simulink model "TST_PIntkVUs_VD"  (R2016b)
settings: Solver=FixedStepDiscrete  StartTime=0.0  StopTime=simTime  FixedStep=sampleTime  RelTol=1e-3
values from neighbouring files (symbols this model uses):
  testCase = 1    [initTST_PIntkVUs_VD_001.m]    (also in initTST_PIntkVUs_VD_002.m = 2; initTST_PIntkVUs_VD_003.m = 3)
libraries: simulink x7, UnitTest_Lib x3
settings Model: Creator=zhengjinyan  LastModifiedBy=zhengjinyan
settings DebuggingCC: SignalRangeChecking=error

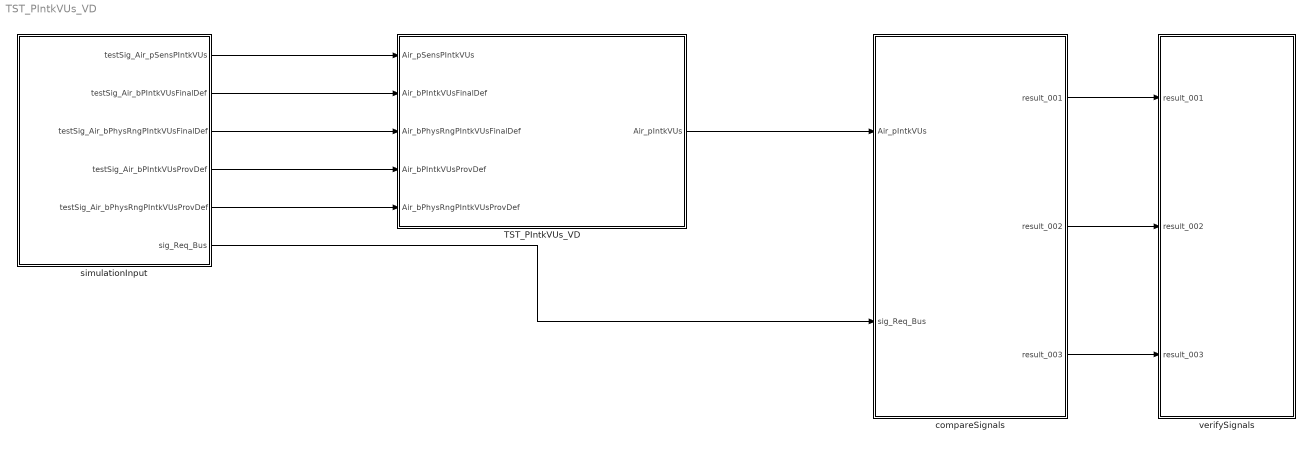
== system TST_PIntkVUs_VD ==
  TST_PIntkVUs_VD : Subsystem
  compareSignals : Subsystem
  simulationInput : Subsystem
  verifySignals : Subsystem
  wires:
  simulationInput/1(testSig_Air_pSensPIntkVUs) -> TST_PIntkVUs_VD/1(Air_pSensPIntkVUs)
  simulationInput/2(testSig_Air_bPIntkVUsFinalDef) -> TST_PIntkVUs_VD/2(Air_bPIntkVUsFinalDef)
  simulationInput/3(testSig_Air_bPhysRngPIntkVUsFinalDef) -> TST_PIntkVUs_VD/3(Air_bPhysRngPIntkVUsFinalDef)
  simulationInput/4(testSig_Air_bPIntkVUsProvDef) -> TST_PIntkVUs_VD/4(Air_bPIntkVUsProvDef)
  simulationInput/5(testSig_Air_bPhysRngPIntkVUsProvDef) -> TST_PIntkVUs_VD/5(Air_bPhysRngPIntkVUsProvDef)
  TST_PIntkVUs_VD/1(Air_pIntkVUs) -> compareSignals/1(Air_pIntkVUs)
  simulationInput/6(sig_Req_Bus) -> compareSignals/2(sig_Req_Bus)
  compareSignals/1(result_001) -> verifySignals/1(result_001)
  compareSignals/2(result_002) -> verifySignals/2(result_002)
  compareSignals/3(result_003) -> verifySignals/3(result_003)

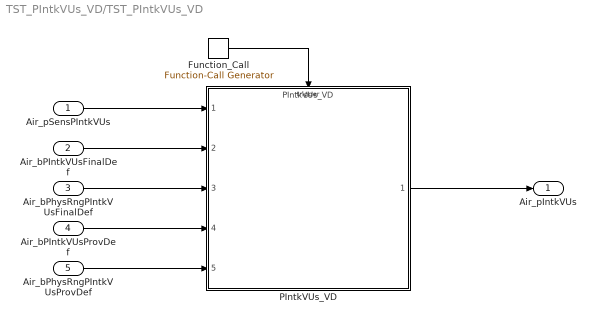
== system TST_PIntkVUs_VD/TST_PIntkVUs_VD ==
  Air_pSensPIntkVUs : Inport
  Air_bPIntkVUsFinalDef : Inport  Port=2
  Air_bPhysRngPIntkVUsFinalDef : Inport  Port=3
  Air_bPIntkVUsProvDef : Inport  Port=4
  Air_bPhysRngPIntkVUsProvDef : Inport  Port=5
  Function_Call : simulink/Ports & Subsystems/Function-Call Generator  sample_time=sampleTime  numberOfIterations=1
  PIntkVUs_VD : ModelReference  ModelNameDialog=PIntkVUs_VD  SimulationMode=Normal  ModelReferenceVersion=1.31  TriggerPortName=function  TriggerPortTriggerType=function-call  TriggerPortStatesWhenEnabling=held
  Air_pIntkVUs : Outport
  wires:
  Function_Call/1 -> PIntkVUs_VD/Trigger
  Air_pSensPIntkVUs/1 -> PIntkVUs_VD/1
  Air_bPIntkVUsFinalDef/1 -> PIntkVUs_VD/2
  Air_bPhysRngPIntkVUsFinalDef/1 -> PIntkVUs_VD/3
  Air_bPIntkVUsProvDef/1 -> PIntkVUs_VD/4
  Air_bPhysRngPIntkVUsProvDef/1 -> PIntkVUs_VD/5
  PIntkVUs_VD/1 -> Air_pIntkVUs/1

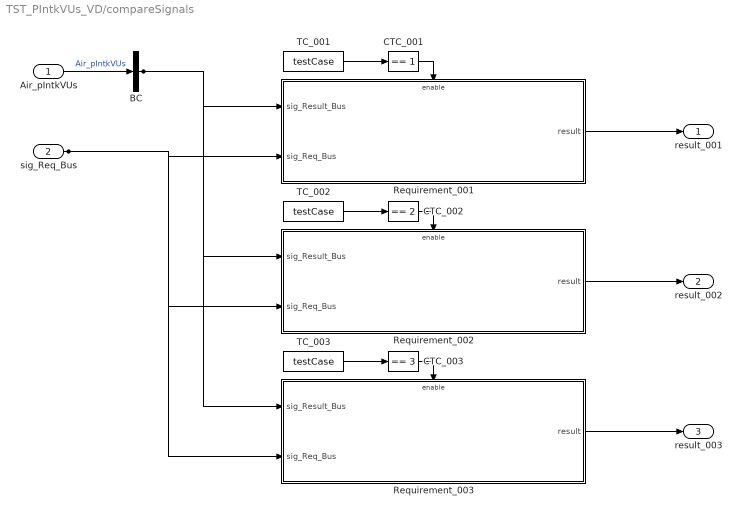
== system TST_PIntkVUs_VD/compareSignals ==
  Air_pIntkVUs : Inport
  sig_Req_Bus : Inport  Port=2
  BC : BusCreator  Inputs=1
  CTC_001 : simulink/Logic and Bit Operations/Compare To Constant  relop===  const=1  OutDataTypeStr=boolean
  CTC_002 : simulink/Logic and Bit Operations/Compare To Constant  relop===  const=2  OutDataTypeStr=boolean
  CTC_003 : simulink/Logic and Bit Operations/Compare To Constant  relop===  const=3  OutDataTypeStr=boolean
  Requirement_001 : Subsystem
  Requirement_002 : Subsystem
  Requirement_003 : Subsystem
  TC_001 : Constant  Value=testCase
  TC_002 : Constant  Value=testCase
  TC_003 : Constant  Value=testCase
  result_001 : Outport
  result_002 : Outport  Port=2
  result_003 : Outport  Port=3
  wires:
  Air_pIntkVUs/1 -> BC/1  "Air_pIntkVUs"
  TC_001/1 -> CTC_001/1
  CTC_001/1 -> Requirement_001/Enable
  sig_Req_Bus/1 -> Requirement_001/2(sig_Req_Bus), Requirement_002/2(sig_Req_Bus), Requirement_003/2(sig_Req_Bus)
  BC/1 -> Requirement_001/1(sig_Result_Bus), Requirement_002/1(sig_Result_Bus), Requirement_003/1(sig_Result_Bus)
  Requirement_001/1(result) -> result_001/1
  TC_002/1 -> CTC_002/1
  CTC_002/1 -> Requirement_002/Enable
  Requirement_002/1(result) -> result_002/1
  TC_003/1 -> CTC_003/1
  CTC_003/1 -> Requirement_003/Enable
  Requirement_003/1(result) -> result_003/1

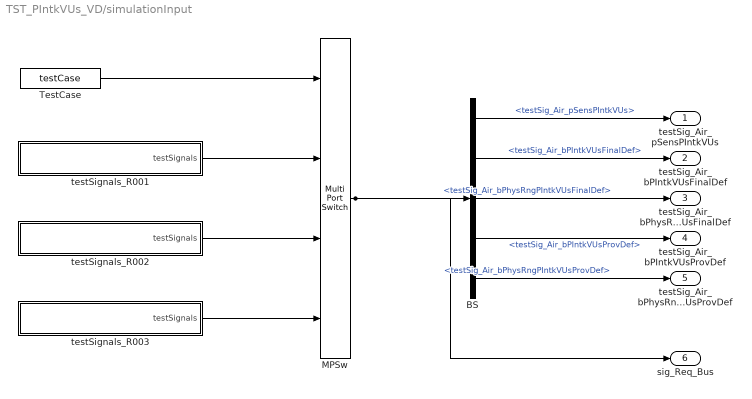
== system TST_PIntkVUs_VD/simulationInput ==
  BS : BusSelector  OutputSignals=testSig_Air_pSensPIntkVUs,testSig_Air_bPIntkVUsFinalDef,testSig_Air_bPhysRngPIntkVUsFinalDef,testSig_Air_bPIntkVUsProvDef,testSig_Air_bPhysRngPIntkVUsProvDef
  MPSw : MultiPortSwitch  SaturateOnIntegerOverflow=on  InputSameDT=on
  TestCase : Constant  Value=testCase
  testSignals_R001 : Subsystem
  testSignals_R002 : Subsystem
  testSignals_R003 : Subsystem
  testSig_Air_pSensPIntkVUs : Outport
  testSig_Air_bPIntkVUsFinalDef : Outport  Port=2
  testSig_Air_bPhysRngPIntkVUsFinalDef : Outport  Port=3
  testSig_Air_bPIntkVUsProvDef : Outport  Port=4
  testSig_Air_bPhysRngPIntkVUsProvDef : Outport  Port=5
  sig_Req_Bus : Outport  Port=6
  wires:
  BS/1 -> testSig_Air_pSensPIntkVUs/1  "<testSig_Air_pSensPIntkVUs>"
  BS/2 -> testSig_Air_bPIntkVUsFinalDef/1  "<testSig_Air_bPIntkVUsFinalDef>"
  BS/3 -> testSig_Air_bPhysRngPIntkVUsFinalDef/1  "<testSig_Air_bPhysRngPIntkVUsFinalDef>"
  BS/4 -> testSig_Air_bPIntkVUsProvDef/1  "<testSig_Air_bPIntkVUsProvDef>"
  BS/5 -> testSig_Air_bPhysRngPIntkVUsProvDef/1  "<testSig_Air_bPhysRngPIntkVUsProvDef>"
  MPSw/1 -> BS/1, sig_Req_Bus/1
  TestCase/1 -> MPSw/1
  testSignals_R001/1(testSignals) -> MPSw/2
  testSignals_R002/1(testSignals) -> MPSw/3
  testSignals_R003/1(testSignals) -> MPSw/4

== system TST_PIntkVUs_VD/verifySignals ==
  result_001 : Inport
  result_002 : Inport  Port=2
  result_003 : Inport  Port=3
  Assertion_001 : Assertion  Enabled=off
  Assertion_002 : Assertion  Enabled=off
  Assertion_003 : Assertion  Enabled=off
  wires:
  result_001/1 -> Assertion_001/1
  result_002/1 -> Assertion_002/1
  result_003/1 -> Assertion_003/1

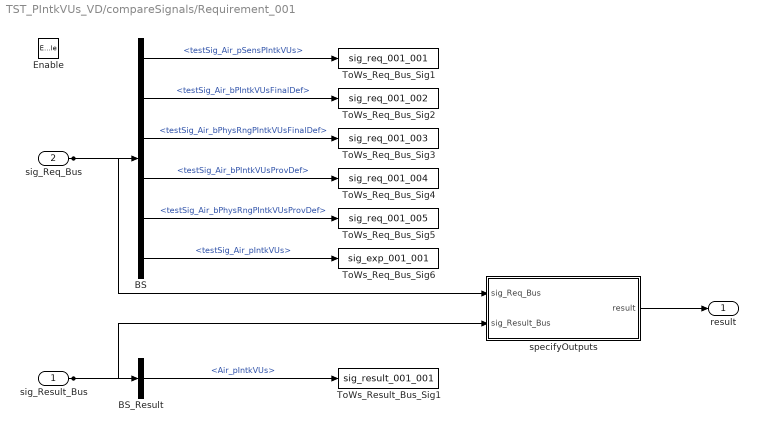
== system TST_PIntkVUs_VD/compareSignals/Requirement_001 ==
  sig_Result_Bus : Inport
  sig_Req_Bus : Inport  Port=2
  Enable : EnablePort
  BS : BusSelector  OutputSignals=testSig_Air_pSensPIntkVUs,testSig_Air_bPIntkVUsFinalDef,testSig_Air_bPhysRngPIntkVUsFinalDef,testSig_Air_bPIntkVUsProvDef,testSig_Air_bPhysRngPIntkVUsProvDef,testSig_Air_pIntkVUs
  BS_Result : BusSelector  OutputSignals=Air_pIntkVUs
  ToWs_Req_Bus_Sig1 : ToWorkspace  VariableName=sig_req_001_001  SaveFormat=Structure With Time
  ToWs_Req_Bus_Sig2 : ToWorkspace  VariableName=sig_req_001_002  SaveFormat=Structure With Time
  ToWs_Req_Bus_Sig3 : ToWorkspace  VariableName=sig_req_001_003  SaveFormat=Structure With Time
  ToWs_Req_Bus_Sig4 : ToWorkspace  VariableName=sig_req_001_004  SaveFormat=Structure With Time
  ToWs_Req_Bus_Sig5 : ToWorkspace  VariableName=sig_req_001_005  SaveFormat=Structure With Time
  ToWs_Req_Bus_Sig6 : ToWorkspace  VariableName=sig_exp_001_001  SaveFormat=Structure With Time
  ToWs_Result_Bus_Sig1 : ToWorkspace  VariableName=sig_result_001_001  SaveFormat=Structure With Time
  specifyOutputs : Subsystem
  result : Outport
  wires:
  sig_Req_Bus/1 -> BS/1, specifyOutputs/1(sig_Req_Bus)
  BS/1 -> ToWs_Req_Bus_Sig1/1  "<testSig_Air_pSensPIntkVUs>"
  BS/2 -> ToWs_Req_Bus_Sig2/1  "<testSig_Air_bPIntkVUsFinalDef>"
  BS/3 -> ToWs_Req_Bus_Sig3/1  "<testSig_Air_bPhysRngPIntkVUsFinalDef>"
  BS/4 -> ToWs_Req_Bus_Sig4/1  "<testSig_Air_bPIntkVUsProvDef>"
  BS/5 -> ToWs_Req_Bus_Sig5/1  "<testSig_Air_bPhysRngPIntkVUsProvDef>"
  BS/6 -> ToWs_Req_Bus_Sig6/1  "<testSig_Air_pIntkVUs>"
  sig_Result_Bus/1 -> BS_Result/1, specifyOutputs/2(sig_Result_Bus)
  BS_Result/1 -> ToWs_Result_Bus_Sig1/1  "<Air_pIntkVUs>"
  specifyOutputs/1(result) -> result/1

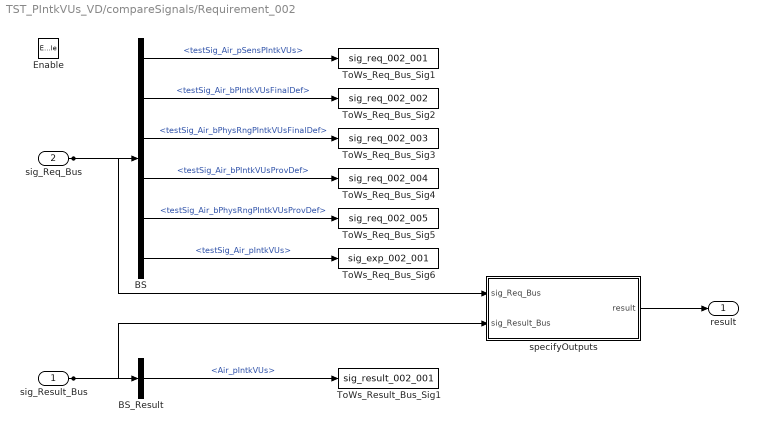
== system TST_PIntkVUs_VD/compareSignals/Requirement_002 ==
  sig_Result_Bus : Inport
  sig_Req_Bus : Inport  Port=2
  Enable : EnablePort
  BS : BusSelector  OutputSignals=testSig_Air_pSensPIntkVUs,testSig_Air_bPIntkVUsFinalDef,testSig_Air_bPhysRngPIntkVUsFinalDef,testSig_Air_bPIntkVUsProvDef,testSig_Air_bPhysRngPIntkVUsProvDef,testSig_Air_pIntkVUs
  BS_Result : BusSelector  OutputSignals=Air_pIntkVUs
  ToWs_Req_Bus_Sig1 : ToWorkspace  VariableName=sig_req_002_001  SaveFormat=Structure With Time
  ToWs_Req_Bus_Sig2 : ToWorkspace  VariableName=sig_req_002_002  SaveFormat=Structure With Time
  ToWs_Req_Bus_Sig3 : ToWorkspace  VariableName=sig_req_002_003  SaveFormat=Structure With Time
  ToWs_Req_Bus_Sig4 : ToWorkspace  VariableName=sig_req_002_004  SaveFormat=Structure With Time
  ToWs_Req_Bus_Sig5 : ToWorkspace  VariableName=sig_req_002_005  SaveFormat=Structure With Time
  ToWs_Req_Bus_Sig6 : ToWorkspace  VariableName=sig_exp_002_001  SaveFormat=Structure With Time
  ToWs_Result_Bus_Sig1 : ToWorkspace  VariableName=sig_result_002_001  SaveFormat=Structure With Time
  specifyOutputs : Subsystem
  result : Outport
  wires:
  sig_Req_Bus/1 -> BS/1, specifyOutputs/1(sig_Req_Bus)
  BS/1 -> ToWs_Req_Bus_Sig1/1  "<testSig_Air_pSensPIntkVUs>"
  BS/2 -> ToWs_Req_Bus_Sig2/1  "<testSig_Air_bPIntkVUsFinalDef>"
  BS/3 -> ToWs_Req_Bus_Sig3/1  "<testSig_Air_bPhysRngPIntkVUsFinalDef>"
  BS/4 -> ToWs_Req_Bus_Sig4/1  "<testSig_Air_bPIntkVUsProvDef>"
  BS/5 -> ToWs_Req_Bus_Sig5/1  "<testSig_Air_bPhysRngPIntkVUsProvDef>"
  BS/6 -> ToWs_Req_Bus_Sig6/1  "<testSig_Air_pIntkVUs>"
  sig_Result_Bus/1 -> BS_Result/1, specifyOutputs/2(sig_Result_Bus)
  BS_Result/1 -> ToWs_Result_Bus_Sig1/1  "<Air_pIntkVUs>"
  specifyOutputs/1(result) -> result/1

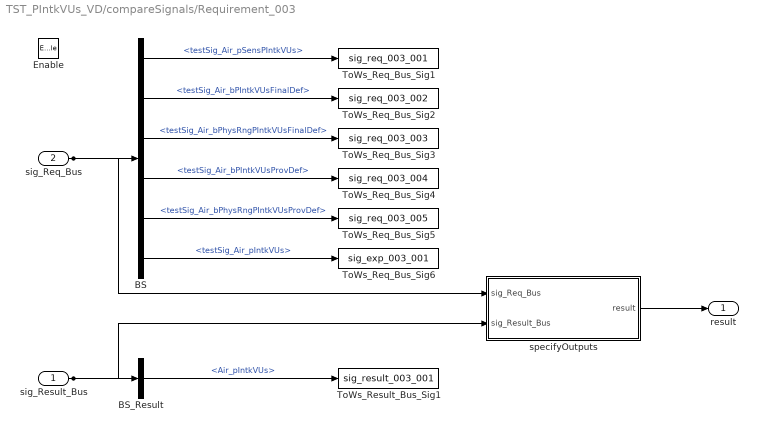
== system TST_PIntkVUs_VD/compareSignals/Requirement_003 ==
  sig_Result_Bus : Inport
  sig_Req_Bus : Inport  Port=2
  Enable : EnablePort
  BS : BusSelector  OutputSignals=testSig_Air_pSensPIntkVUs,testSig_Air_bPIntkVUsFinalDef,testSig_Air_bPhysRngPIntkVUsFinalDef,testSig_Air_bPIntkVUsProvDef,testSig_Air_bPhysRngPIntkVUsProvDef,testSig_Air_pIntkVUs
  BS_Result : BusSelector  OutputSignals=Air_pIntkVUs
  ToWs_Req_Bus_Sig1 : ToWorkspace  VariableName=sig_req_003_001  SaveFormat=Structure With Time
  ToWs_Req_Bus_Sig2 : ToWorkspace  VariableName=sig_req_003_002  SaveFormat=Structure With Time
  ToWs_Req_Bus_Sig3 : ToWorkspace  VariableName=sig_req_003_003  SaveFormat=Structure With Time
  ToWs_Req_Bus_Sig4 : ToWorkspace  VariableName=sig_req_003_004  SaveFormat=Structure With Time
  ToWs_Req_Bus_Sig5 : ToWorkspace  VariableName=sig_req_003_005  SaveFormat=Structure With Time
  ToWs_Req_Bus_Sig6 : ToWorkspace  VariableName=sig_exp_003_001  SaveFormat=Structure With Time
  ToWs_Result_Bus_Sig1 : ToWorkspace  VariableName=sig_result_003_001  SaveFormat=Structure With Time
  specifyOutputs : Subsystem
  result : Outport
  wires:
  sig_Req_Bus/1 -> BS/1, specifyOutputs/1(sig_Req_Bus)
  BS/1 -> ToWs_Req_Bus_Sig1/1  "<testSig_Air_pSensPIntkVUs>"
  BS/2 -> ToWs_Req_Bus_Sig2/1  "<testSig_Air_bPIntkVUsFinalDef>"
  BS/3 -> ToWs_Req_Bus_Sig3/1  "<testSig_Air_bPhysRngPIntkVUsFinalDef>"
  BS/4 -> ToWs_Req_Bus_Sig4/1  "<testSig_Air_bPIntkVUsProvDef>"
  BS/5 -> ToWs_Req_Bus_Sig5/1  "<testSig_Air_bPhysRngPIntkVUsProvDef>"
  BS/6 -> ToWs_Req_Bus_Sig6/1  "<testSig_Air_pIntkVUs>"
  sig_Result_Bus/1 -> BS_Result/1, specifyOutputs/2(sig_Result_Bus)
  BS_Result/1 -> ToWs_Result_Bus_Sig1/1  "<Air_pIntkVUs>"
  specifyOutputs/1(result) -> result/1

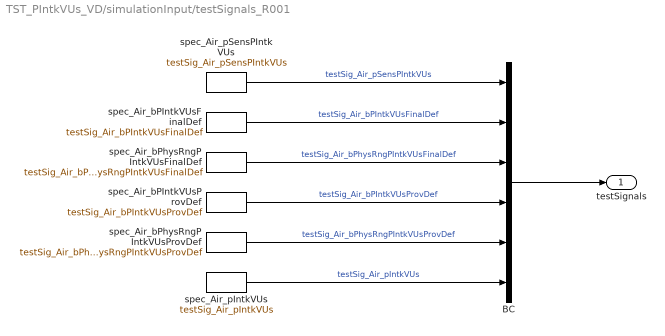
== system TST_PIntkVUs_VD/simulationInput/testSignals_R001 ==
  BC : BusCreator  Inputs=6
  spec_Air_bPIntkVUsFinalDef : FromWorkspace  VariableName=testSig_Air_bPIntkVUsFinalDef  Interpolate=off  OutputAfterFinalValue=Holding final value
  spec_Air_bPIntkVUsProvDef : FromWorkspace  VariableName=testSig_Air_bPIntkVUsProvDef  Interpolate=off  OutputAfterFinalValue=Holding final value
  spec_Air_bPhysRngPIntkVUsFinalDef : FromWorkspace  VariableName=testSig_Air_bPhysRngPIntkVUsFinalDef  Interpolate=off  OutputAfterFinalValue=Holding final value
  spec_Air_bPhysRngPIntkVUsProvDef : FromWorkspace  VariableName=testSig_Air_bPhysRngPIntkVUsProvDef  Interpolate=off  OutputAfterFinalValue=Holding final value
  spec_Air_pIntkVUs : FromWorkspace  VariableName=testSig_Air_pIntkVUs  Interpolate=off  OutputAfterFinalValue=Holding final value
  spec_Air_pSensPIntkVUs : FromWorkspace  VariableName=testSig_Air_pSensPIntkVUs  Interpolate=off  OutputAfterFinalValue=Holding final value
  testSignals : Outport
  wires:
  BC/1 -> testSignals/1
  spec_Air_pSensPIntkVUs/1 -> BC/1  "testSig_Air_pSensPIntkVUs"
  spec_Air_bPIntkVUsFinalDef/1 -> BC/2  "testSig_Air_bPIntkVUsFinalDef"
  spec_Air_bPhysRngPIntkVUsFinalDef/1 -> BC/3  "testSig_Air_bPhysRngPIntkVUsFinalDef"
  spec_Air_bPIntkVUsProvDef/1 -> BC/4  "testSig_Air_bPIntkVUsProvDef"
  spec_Air_bPhysRngPIntkVUsProvDef/1 -> BC/5  "testSig_Air_bPhysRngPIntkVUsProvDef"
  spec_Air_pIntkVUs/1 -> BC/6  "testSig_Air_pIntkVUs"

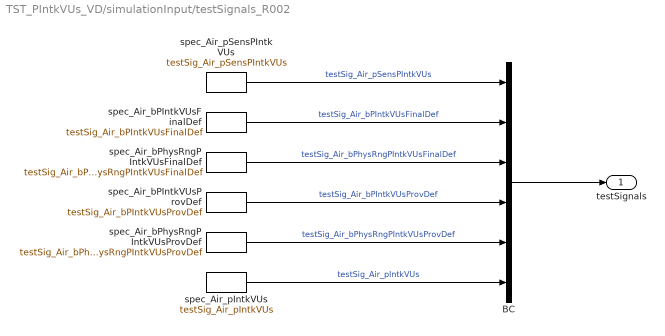
== system TST_PIntkVUs_VD/simulationInput/testSignals_R002 ==
  BC : BusCreator  Inputs=6
  spec_Air_bPIntkVUsFinalDef : FromWorkspace  VariableName=testSig_Air_bPIntkVUsFinalDef  Interpolate=off  OutputAfterFinalValue=Holding final value
  spec_Air_bPIntkVUsProvDef : FromWorkspace  VariableName=testSig_Air_bPIntkVUsProvDef  Interpolate=off  OutputAfterFinalValue=Holding final value
  spec_Air_bPhysRngPIntkVUsFinalDef : FromWorkspace  VariableName=testSig_Air_bPhysRngPIntkVUsFinalDef  Interpolate=off  OutputAfterFinalValue=Holding final value
  spec_Air_bPhysRngPIntkVUsProvDef : FromWorkspace  VariableName=testSig_Air_bPhysRngPIntkVUsProvDef  Interpolate=off  OutputAfterFinalValue=Holding final value
  spec_Air_pIntkVUs : FromWorkspace  VariableName=testSig_Air_pIntkVUs  Interpolate=off  OutputAfterFinalValue=Holding final value
  spec_Air_pSensPIntkVUs : FromWorkspace  VariableName=testSig_Air_pSensPIntkVUs  Interpolate=off  OutputAfterFinalValue=Holding final value
  testSignals : Outport
  wires:
  BC/1 -> testSignals/1
  spec_Air_pSensPIntkVUs/1 -> BC/1  "testSig_Air_pSensPIntkVUs"
  spec_Air_bPIntkVUsFinalDef/1 -> BC/2  "testSig_Air_bPIntkVUsFinalDef"
  spec_Air_bPhysRngPIntkVUsFinalDef/1 -> BC/3  "testSig_Air_bPhysRngPIntkVUsFinalDef"
  spec_Air_bPIntkVUsProvDef/1 -> BC/4  "testSig_Air_bPIntkVUsProvDef"
  spec_Air_bPhysRngPIntkVUsProvDef/1 -> BC/5  "testSig_Air_bPhysRngPIntkVUsProvDef"
  spec_Air_pIntkVUs/1 -> BC/6  "testSig_Air_pIntkVUs"

== system TST_PIntkVUs_VD/simulationInput/testSignals_R003 ==
  BC : BusCreator  Inputs=6
  spec_Air_bPIntkVUsFinalDef : FromWorkspace  VariableName=testSig_Air_bPIntkVUsFinalDef  Interpolate=off  OutputAfterFinalValue=Holding final value
  spec_Air_bPIntkVUsProvDef : FromWorkspace  VariableName=testSig_Air_bPIntkVUsProvDef  Interpolate=off  OutputAfterFinalValue=Holding final value
  spec_Air_bPhysRngPIntkVUsFinalDef : FromWorkspace  VariableName=testSig_Air_bPhysRngPIntkVUsFinalDef  Interpolate=off  OutputAfterFinalValue=Holding final value
  spec_Air_bPhysRngPIntkVUsProvDef : FromWorkspace  VariableName=testSig_Air_bPhysRngPIntkVUsProvDef  Interpolate=off  OutputAfterFinalValue=Holding final value
  spec_Air_pIntkVUs : FromWorkspace  VariableName=testSig_Air_pIntkVUs  Interpolate=off  OutputAfterFinalValue=Holding final value
  spec_Air_pSensPIntkVUs : FromWorkspace  VariableName=testSig_Air_pSensPIntkVUs  Interpolate=off  OutputAfterFinalValue=Holding final value
  testSignals : Outport
  wires:
  BC/1 -> testSignals/1
  spec_Air_pSensPIntkVUs/1 -> BC/1  "testSig_Air_pSensPIntkVUs"
  spec_Air_bPIntkVUsFinalDef/1 -> BC/2  "testSig_Air_bPIntkVUsFinalDef"
  spec_Air_bPhysRngPIntkVUsFinalDef/1 -> BC/3  "testSig_Air_bPhysRngPIntkVUsFinalDef"
  spec_Air_bPIntkVUsProvDef/1 -> BC/4  "testSig_Air_bPIntkVUsProvDef"
  spec_Air_bPhysRngPIntkVUsProvDef/1 -> BC/5  "testSig_Air_bPhysRngPIntkVUsProvDef"
  spec_Air_pIntkVUs/1 -> BC/6  "testSig_Air_pIntkVUs"

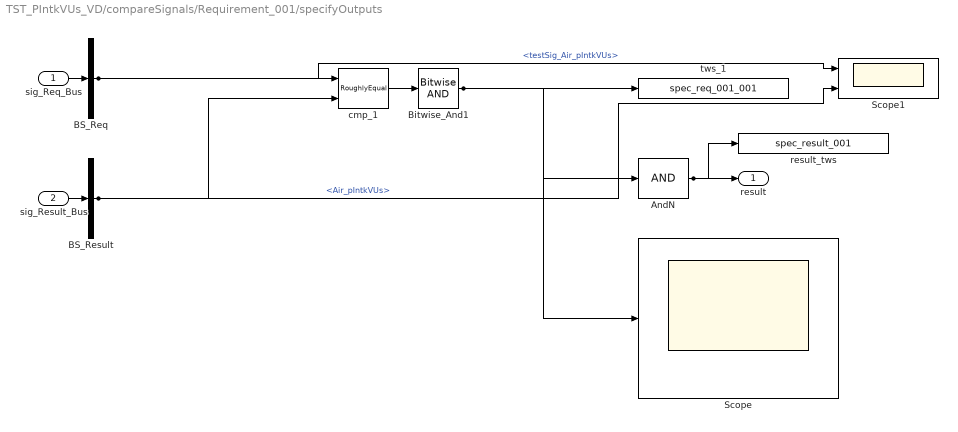
== system TST_PIntkVUs_VD/compareSignals/Requirement_001/specifyOutputs ==
  sig_Req_Bus : Inport
  sig_Result_Bus : Inport  Port=2
  AndN : Logic  Inputs=1
  BS_Req : BusSelector  OutputSignals=testSig_Air_pIntkVUs
  BS_Result : BusSelector  OutputSignals=Air_pIntkVUs
  Bitwise_And1 : simulink/Logic and Bit Operations/Bitwise Operator  logicop=AND  UseBitMask=off  BitMask=bin2dec('11011001')  BitMaskRealWorld=Stored Integer
  Scope : Scope
  Scope1 : Scope  NumInputPorts=2
  cmp_1 : UnitTest_Lib/RoughlyEqual  slope=0.1
  result_tws : ToWorkspace  VariableName=spec_result_001
  tws_1 : ToWorkspace  VariableName=spec_req_001_001
  result : Outport
  wires:
  sig_Req_Bus/1 -> BS_Req/1
  sig_Result_Bus/1 -> BS_Result/1
  AndN/1 -> result/1, result_tws/1
  BS_Req/1 -> cmp_1/1, Scope1/1  "<testSig_Air_pIntkVUs>"
  BS_Result/1 -> cmp_1/2, Scope1/2  "<Air_pIntkVUs>"
  cmp_1/1 -> Bitwise_And1/1
  Bitwise_And1/1 -> tws_1/1, AndN/1, Scope/1

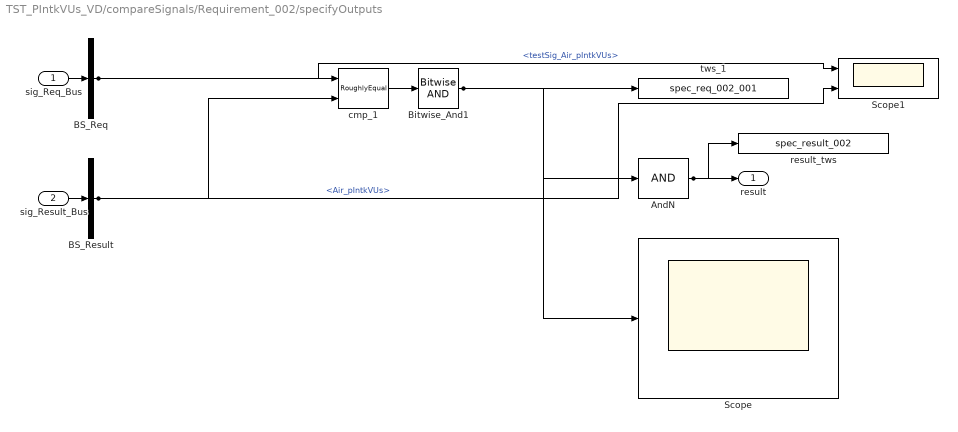
== system TST_PIntkVUs_VD/compareSignals/Requirement_002/specifyOutputs ==
  sig_Req_Bus : Inport
  sig_Result_Bus : Inport  Port=2
  AndN : Logic  Inputs=1
  BS_Req : BusSelector  OutputSignals=testSig_Air_pIntkVUs
  BS_Result : BusSelector  OutputSignals=Air_pIntkVUs
  Bitwise_And1 : simulink/Logic and Bit Operations/Bitwise Operator  logicop=AND  UseBitMask=off  BitMask=bin2dec('11011001')  BitMaskRealWorld=Stored Integer
  Scope : Scope
  Scope1 : Scope  NumInputPorts=2
  cmp_1 : UnitTest_Lib/RoughlyEqual  slope=0.1
  result_tws : ToWorkspace  VariableName=spec_result_002
  tws_1 : ToWorkspace  VariableName=spec_req_002_001
  result : Outport
  wires:
  sig_Req_Bus/1 -> BS_Req/1
  sig_Result_Bus/1 -> BS_Result/1
  AndN/1 -> result/1, result_tws/1
  BS_Req/1 -> cmp_1/1, Scope1/1  "<testSig_Air_pIntkVUs>"
  BS_Result/1 -> cmp_1/2, Scope1/2  "<Air_pIntkVUs>"
  cmp_1/1 -> Bitwise_And1/1
  Bitwise_And1/1 -> tws_1/1, AndN/1, Scope/1

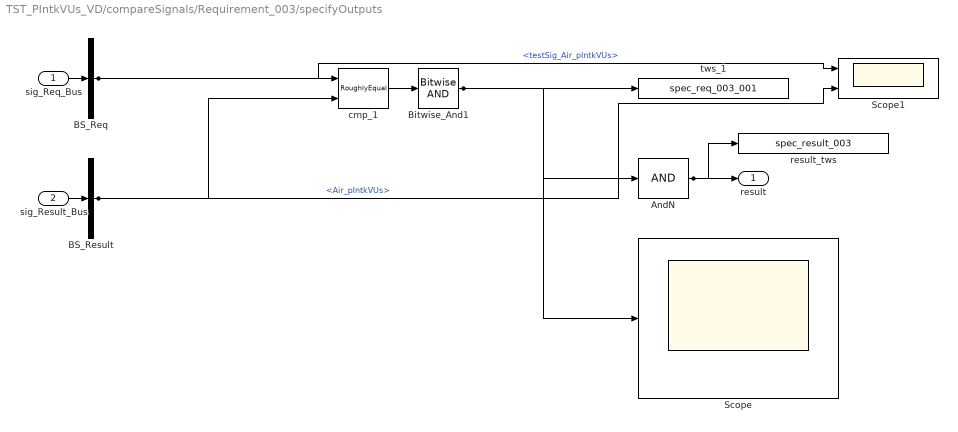
== system TST_PIntkVUs_VD/compareSignals/Requirement_003/specifyOutputs ==
  sig_Req_Bus : Inport
  sig_Result_Bus : Inport  Port=2
  AndN : Logic  Inputs=1
  BS_Req : BusSelector  OutputSignals=testSig_Air_pIntkVUs
  BS_Result : BusSelector  OutputSignals=Air_pIntkVUs
  Bitwise_And1 : simulink/Logic and Bit Operations/Bitwise Operator  logicop=AND  UseBitMask=off  BitMask=bin2dec('11011001')  BitMaskRealWorld=Stored Integer
  Scope : Scope
  Scope1 : Scope  NumInputPorts=2
  cmp_1 : UnitTest_Lib/RoughlyEqual  slope=0.1
  result_tws : ToWorkspace  VariableName=spec_result_003
  tws_1 : ToWorkspace  VariableName=spec_req_003_001
  result : Outport
  wires:
  sig_Req_Bus/1 -> BS_Req/1
  sig_Result_Bus/1 -> BS_Result/1
  AndN/1 -> result/1, result_tws/1
  BS_Req/1 -> cmp_1/1, Scope1/1  "<testSig_Air_pIntkVUs>"
  BS_Result/1 -> cmp_1/2, Scope1/2  "<Air_pIntkVUs>"
  cmp_1/1 -> Bitwise_And1/1
  Bitwise_And1/1 -> tws_1/1, AndN/1, Scope/1
